simulink model "Lab_3_Simulink"  (R2023b)
settings: Solver=VariableStepAuto  StartTime=0.0  StopTime=inf  RelTol=1e-3
undefined symbols (not defined in the file or in its folder): CR, DiscIntNeverNeededParam, LF
libraries: instrumentseriallib x3
settings Model: Creator=blake  LastModifiedBy=blake

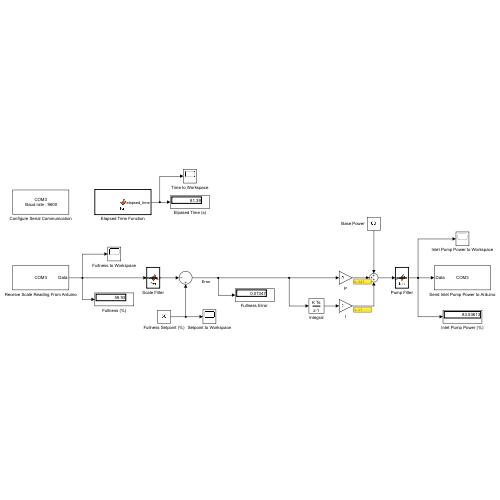
[thumbnail: Simulink's stored preview of the top-level diagram]
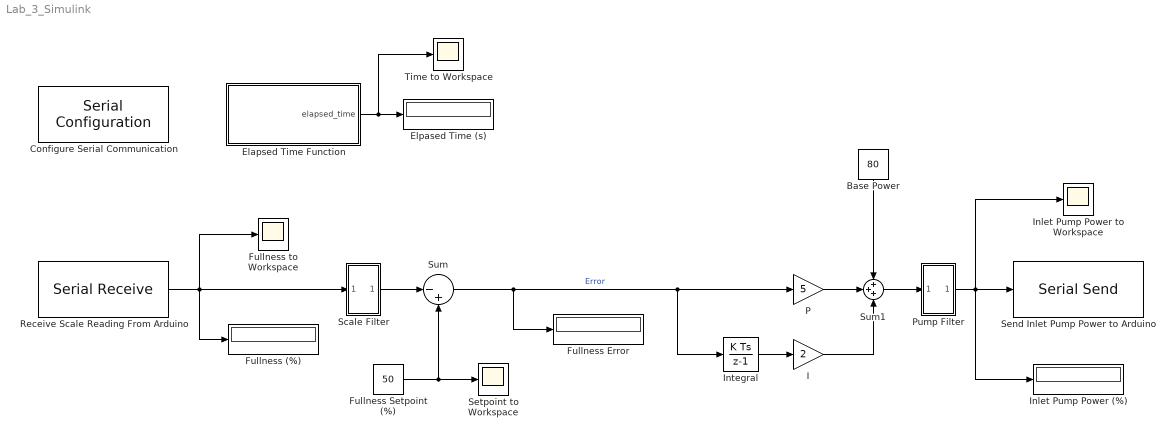
== system Lab_3_Simulink ==
  Base Power : Constant  Value=80
  Configure Serial Communication : instrumentseriallib/Serial Configuration  Priority=-200000  PortSel=COM3  Port=COM3  ComPort=COM3  BaudRate=9600  DataBits=8  Parity=none  StopBits=1  ByteOrder=little-endian  FlowControl=none  Timeout=2  SimulateUsing=Interpreted execution  BlockInModel=on  aMode=1
  Elapsed Time Function : MATLAB Function  TreatAsAtomicUnit=on
  Elpased Time (s) : Display
  Fullness (%) : Display
  "Fullness Error " : Display
  Fullness Setpoint (%) : Constant  Value=50
  Fullness to Workspace : Scope
  I : Gain  Gain=2
  Inlet Pump Power (%) : Display
  Inlet Pump Power to Workspace : Scope
  Integral : DiscreteIntegrator  SampleTime=-1  ICPrevOutput=DiscIntNeverNeededParam  ICPrevScaledInput=DiscIntNeverNeededParam
  P : Gain  Gain=5
  Pump Filter : MATLAB Function  TreatAsAtomicUnit=on
  Receive Scale Reading From Arduino : instrumentseriallib/Serial Receive  Priority=1  PortSel=COM3  Port=COM3  ComPort=COM3  DataType=single  SaveDataType=uint8  ToggleHeader=off  Header=[]  DataSize=1  ToggleTerminator=on  Terminator=CR/LF ('\r\n')  CustomTerminator=[]  InputFormat=Column major  ToggleDataSize=on  EnableBlockingMode=on  ActionDataUnavailable=Output last received value  ActionWhenDataUnavailable=Output last received value  CustomValue=0  SampleTime=0.05  SimulateUsing=Interpreted execution  BlockInModel=on  aMode=1
  Scale Filter : MATLAB Function  TreatAsAtomicUnit=on
  Send Inlet Pump Power to Arduino : instrumentseriallib/Serial Send  Priority=1  PortSel=COM3  Port=COM3  ComPort=COM3  Header=[]  Terminator=CR/LF ('\r\n')  CustomTerminator=[]  EnableBlockingMode=on  SimulateUsing=Interpreted execution  BlockInModel=on  aMode=1
  Setpoint to Workspace : Scope
  Sum : Sum  Inputs=|-+
  Sum1 : Sum  Inputs=+++
  Time to Workspace : Scope
  wires:
  Elapsed Time Function/1(elapsed_time) -> Elpased Time (s)/1, Time to Workspace/1
  Sum/1 -> Integral/1, P/1, "Fullness Error "/1  "Error"
  Receive Scale Reading From Arduino/1 -> Fullness to Workspace/1, Scale Filter/1(scale_reading), Fullness (%)/1
  Pump Filter/1(filtered_power) -> Inlet Pump Power to Workspace/1, Send Inlet Pump Power to Arduino/1, Inlet Pump Power (%)/1
  Fullness Setpoint (%)/1 -> Sum/2, Setpoint to Workspace/1
  Integral/1 -> I/1
  I/1 -> Sum1/3
  P/1 -> Sum1/2
  Base Power/1 -> Sum1/1
  Scale Filter/1(filtered_reading) -> Sum/1
  Sum1/1 -> Pump Filter/1(power)

== matlab function Lab_3_Simulink/Elapsed Time Function ==
  data: elapsed_time output
function elapsed_time = fcn()
    persistent startTime; % persistent variable to store the start time
    
    if isempty(startTime) % check if start_time is empty
        startTime = now;  % initialize start_time with the current time
    end
    
    elapsedDays = now - startTime; % calculate elapsed time in days since start_time
    
    elapsed_time = elapsedDays * 86400; %  convert elapsed time from days to seconds
end

== matlab function Lab_3_Simulink/Pump Filter ==
  data: filtered_power output; power input
function filtered_power = fcn(power)
    if power > 100
        filtered_power = single(100);
    elseif power < 0
        filtered_power = single(0);
    else
        filtered_power = single(power);
    end
end

== matlab function Lab_3_Simulink/Scale Filter ==
  data: filtered_reading output; scale_reading input
function filtered_reading = fcn(scale_reading)
    persistent last_value; % persistent variable to store the start time
    
    if isempty(last_value) % check if start_time is empty
        last_value = single(50);  % initialize start_time with the current time
    end
    
    if scale_reading < 0 || scale_reading > 100
        filtered_reading = last_value;
    else
        filtered_reading = scale_reading;
        last_value = scale_reading;
    end
end
